simulink model "relative_position_sim"  (R2019a)
settings: Solver=VariableStepAuto  StartTime=0.0  StopTime=10.0  RelTol=1e-3
settings Model: Creator=hanabusa  LastModifiedBy=hanabusa

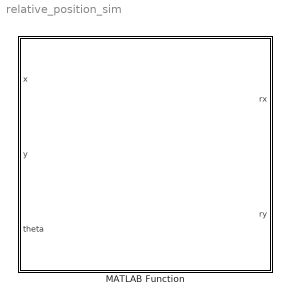
== system relative_position_sim ==
  MATLAB Function : MATLAB Function  TreatAsAtomicUnit=on

== matlab function relative_position_sim/MATLAB Function ==
  data: x input; rx output; y input; theta input; ry output
function [rx,ry]=relative_position(x,y,theta)
N=5;
 for i=1:N
     for j=1:N
       rx(i,j)=cos(theta(i))*(x(j)-x(i))+sin(theta(i))*(y(j)-y(i)); %iから見たjの相対位置
       ry(i,j)=-sin(theta(i))*(x(j)-x(i))+cos(theta(i))*(y(j)-y(i));
     end
 end
end
